simulink model "sm_wing_landing_gear"  (R2021b)
settings: Solver=ode45  StartTime=0  StopTime=10  RelTol=1e-4  AbsTol=1e-4  EnableMultiTasking=on
model workspace (MAT data in the model file):
  ddgrey = [0.15 0.15 0.15]
  dgrey = [0.3 0.3 0.3]
  grey = [0.5 0.5 0.5]
  lgrey = [0.7 0.7 0.7]
  rho_alum = 2700
undefined symbols (not defined in the file): sigbuilder_block, X, Y, Z
libraries: sm_lib x59, sm_wing_landing_gear_lib x45, nesl_utility x7, simulink x2
(part 1 of 3)
Description:
  | Airplane Wing Landing Gear
  | 
  | This model shows a wing landing gear mechanism that can deploy
  | and retract based on the input deploy signal. The mechanism consists
  | of the main column that houses the wheel assembly and the locking
  | mechanism that is used to lock the landing gear in the deployed
  | position.
  | 
  | The mechanism is controlled by two low level controllers (one for
  | deploying and retracting the main column and the other  to lock and
  | unlock the main column into position) and a master controller that
  | coordinates them. The low level controllers are both simple PID
  | controllers. The master controller turns on the deploy/retract
  | controller to deploy the landing gear and when the main column is
  | close enough to the deployed position, it disables the deploy/retract
  |  controller and uses the locking controller to lock the mechanism
  | into position. The reverse happens during retraction.
settings Model: Creator=The MathWorks, Inc.  LastModifiedBy=The MathWorks, Inc.
settings SolverCC: AutoScaleAbsTol=off  AlgebraicLoopSolver=TrustRegion
settings DataIOCC: LimitDataPoints=on  SaveFormat=Array  ReturnWorkspaceOutputs=off
settings OptimizationCC: OptimizeBlockIOStorage=off  BufferReuse=off  GlobalBufferReuse=off  ExpressionFolding=off  ExpressionDepthLimit=2147483647  LocalBlockOutputs=off  LifeSpan=inf  OptimizeDataStoreBuffers=off  BusAssignmentInplaceUpdate=off
settings DebuggingCC: UnderspecifiedInitializationDetection=Classic  MergeDetectMultiDrivingBlocksExec=none  ParameterPrecisionLossMsg=none  FcnCallInpInsideContextMsg=warning  AllowSymbolicDim=off  StateNameClashWarn=warning  SFUnexpectedBacktrackingDiag=warning  SFNoUnconditionalDefaultTransitionDiag=warning  SFExecutionAtInitializationDiag=none  SFMachineParentedDataDiag=warning  ArithmeticOperatorsInVariantConditions=warning
settings HardwareCC: ProdBitPerPointer=32  ProdBitPerSizeT=32  ProdBitPerPtrDiffT=32  ProdLargestAtomicFloat=None  ProdIntDivRoundTo=Undefined  ProdEndianess=Unspecified  ProdWordSize=32  ProdHWDeviceType=32-bit Generic
settings ModelReferenceCC: PropagateSignalLabelsOutOfModel=off
settings SFSimCC: SimUseLocalCustomCode=off  CustomCodeUndefinedFunction=UseInterfaceOnly
settings RTWCC: RTWUseLocalCustomCode=off
settings CodeAppCC: StateflowObjectComments=on
settings GRTTargetCC: TargetLangStandard=C89/C90 (ANSI)  CombineOutputUpdateFcns=off  GRTInterface=on
settings ConfigComp: CovMetricSettings=dw  CovSaveCumulativeToWorkspaceVar=on  CovSaveSingleToWorkspaceVar=on  CovExternalEMLEnable=off  CovSFcnEnable=off
settings SimscapeCC: SimscapeNormalizeSystem=off
settings ConfigurationSet: Description=SimMechanics 2G
settings ExplorerConfigSet: InternalSimMechanicsExplorerSettings="<ExplorerConfiguration><canonicalview>default</canonicalview><AnimationSetting><BasePlaybackSpeed>1.0</BasePlaybackSpeed><PlaybackSpeedFactor>1.0</PlaybackSpeedFactor></AnimationSetting><TilePanel><TileInfo><Tiles Columns=\"1\" Count=\"1\" Rows=\"1\"><Column Left=\"2\" Weight=\"1\"/><Column Left=\"642\"/><Row Top=\"2\" Weight=\"1\"/><Row Top=\"563\"/><Tile Height=\"1\" Width=\"1\" X=\"0\" Y=\"0\"/></Tiles></TileInfo><SceneInfo><SceneViewer><BGColor><R>0.60000002384185791</R><G>0.60000002384185791</G><B>0.60000002384185791</B></BGColor><Camera><Position><X>5.05242413843680716</X><Y>-3.63242412174750484</Y><Z>3.34347951973487101</Z></Position><Center><X>1.82500004768371582</X><Y>-0.405000030994415283</Y><Z>0.116055428981781006</Z></Center><Up><X>-0.408248290463863073</X><Y>0.408248290463863073</Y><Z>0.816496580927726145</Z></Up><Left>-2.13829092979431179</Left><Right>2.13829092979431179</Right><Bottom>-1.76270043253898634</Bottom><Top>1.76270043253898634</Top></Camera></SceneViewer></SceneInfo></TilePanel></ExplorerConfiguration>"

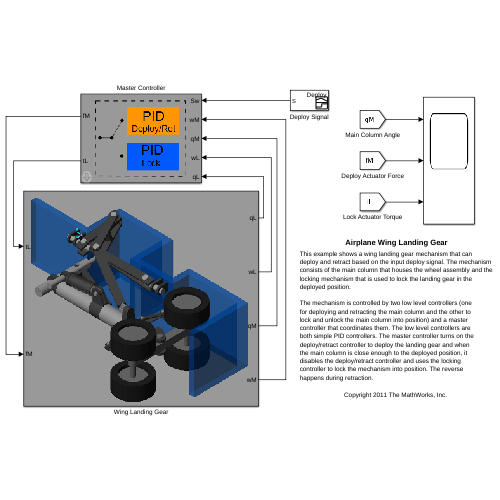
[thumbnail: Simulink's stored preview of the top-level diagram]
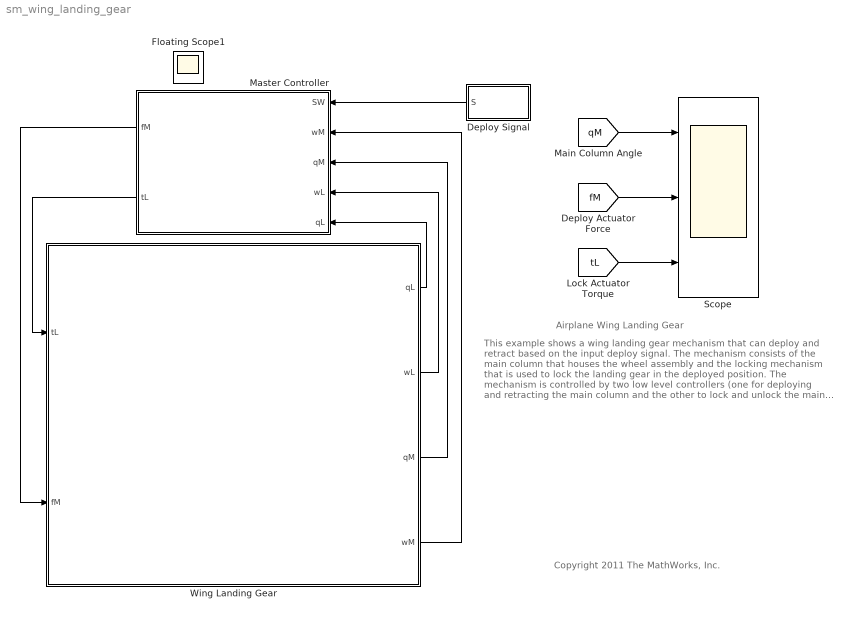
== system sm_wing_landing_gear ==
  note: Airplane Wing Landing Gear
  note: Copyright 2011 The MathWorks, Inc.
  note: This example shows a wing landing gear mechanism that can
      | deploy and retract based on the input deploy signal. The mechanism
      | consists of the main column that houses the wheel assembly and the
      | locking mechanism that is used to lock the landing gear in the
      | deployed position.
      |
      | The mechanism is controlled by two low level controllers (one
      | for deploying and retracting the main column and the other to
      | lock and unlock the main column into position) and a master
      | controller that coordinates them. The low level controllers are
      | both simple PID controllers. The master controller turns on the
      | deploy/retract controller to deploy the landing gear and when
      | the main column is close enough to the deployed position, it
      | disables the deploy/retract controller and uses the locking
      | controller to lock the mechanism into position. The reverse
      | happens during retraction.
  Deploy Signal : Subsystem  Tag=STV Subsys  LoadFcn=sigbuilder_block('load');  StartFcn=sigbuilder_block('start');  StopFcn=sigbuilder_block('stop');  ClipboardFcn=sigbuilder_block('clipboard');  mask(Sigbuilder block){tuvar=[0:10]}
      mask help: Simulink:masks:SigbuilderBlock_MD
      mask init:
      | if ~strcmp(get_param(bdroot(gcbh),'SimulationStatus'),'stopped') tuvar = sigbuilder_block('maskInit'); end
      settings: CopyFcn=sigbuilder_block('copy');  DeleteFcn=sigbuilder_block('delete');  ModelCloseFcn=sigbuilder_block('modelClose');  PreSaveFcn=sigbuilder_block('preSave');  PauseFcn=sigbuilder_block('pause');  ContinueFcn=sigbuilder_block('continue');  NameChangeFcn=sigbuilder_block('namechange');  OpenFcn=sigbuilder_block('open',[387.2 208 550.4 400 ]);  CloseFcn=sigbuilder_block('close');
      mask Display: plot(0, 0, 100, 100,[2, 2, 32, 32, 2], [68, 8, 8, 68, 68],[32, 2], [38, 38], [32, 19, 2],[53, 60, 44], [32, 17, 17, 2],[16, 16, 31, 31]);txt = getActiveGroup(gcbh);text(2, 100, txt,'verticalAlignment', 'top');
  Master Controller : Subsystem  mask(Controller){Kpd=2e5, Kdd=5e4, Kid=10, Kpl=4, Kdl=1, Kil=0.5, qL=5, qUL=1}
      mask prompts: Kpd "Proportional Gain"; Kdd "Derivative Gain"; Kid "Integral Gain"; Kpl "Proportional Gain"; Kdl "Derivative Gain"; Kil "Integral Gain"; qL "Locking Start Angle (deg)"; qUL "Unlocking End Angle (deg)"
      mask help: The mechanism is controlled by two low level controllers (one for deploying and retracting the main column and the other to lock and unlock the main column into position) and a master controller that coordinates them. The low level controllers are both simple PID controllers. The master controller turns on the Deploy/Retract controller which moves the main column into the vertical position. When the angle of the main column is within a certain value of the vertical position (Locking Start Angle specified below), the Locking controller is enabled and the Deploy/Retract Controller is disabled. The Locking controller makes the locking links fully stretched leaving the mechanism in a locked position. During retraction the Locking controller makes the locking links to be bent and starts to lift the main column. Once the main column angle is more than a certain value from the vertical position (Unlocking End Angle specified below), the Locking controller is disabled and the Deploy/Retract controller is enabled, which moves the main column to the horizontal position.
      mask DialogControl ParameterTabVar0 Prompt: Deploy Ctrl
      mask DialogControl ParameterTabVar01 Prompt: Lock Ctrl
      mask DialogControl ParameterTabVar012 Prompt: Master Ctrl
      mask Display:
      | image('sm_wlandgear_controller.png');
      | port_label('input',1,'Sw');
      | port_label('input',2,'wM');
      | port_label('input',3,'qM');
      | port_label('input',4,'wL');
      | port_label('input',5,'qL');
      | port_label('output',2,'tL');
      | port_label('output',1,'fM');
  Scope : Scope  NumInputPorts=3
  Wing Landing Gear : Subsystem
      mask Display:
      | image('sm_wlandgear_plant.png');
      | port_label('output',1,'qL');
      | port_label('output',2,'wL');
      | port_label('output',3,'qM');
      | port_label('output',4,'wM');
      | port_label('input',2,'fM');
      | port_label('input',1,'tL');
  Floating Scope1 : Scope
  wires:
  Deploy Signal/1(S) -> Master Controller/1(SW)
  [tL] -> Scope/3
  [fM] -> Scope/2
  [qM] -> Scope/1
  Wing Landing Gear/1(qL) -> Master Controller/5(qL)
  Wing Landing Gear/2(wL) -> Master Controller/4(wL)
  Wing Landing Gear/3(qM) -> Master Controller/3(qM)
  Wing Landing Gear/4(wM) -> Master Controller/2(wM)
  Master Controller/1(fM) -> Wing Landing Gear/2(fM)
  Master Controller/2(tL) -> Wing Landing Gear/1(tL)

== system sm_wing_landing_gear/Deploy Signal ==
  Demux : Demux  Tag=STV Demux  Outputs=1
      settings: DisplayOption=none
  FromWs : FromWorkspace  Tag=STV FromWs  VariableName=tuvar
      SigBuilderData=|
      | common.afterFinalStr = 'Extrapolate'
      | common.sampleTime = '0'
      | dataSet.timeRange = [0 15]
      | dataSet.name = 'Deploy'
      | sbobj.Groups.Name = 'Deploy'
      | sbobj.Groups.Signals.Name = 'S'
      | sbobj.Groups.Signals.XData = [0 1 1 6 6 15]
      | sbobj.Groups.Signals.YData = [0 0 1 1 0 0]
      | sbobj.Groups.TimeRange = [0 15]
  S : Outport  Tag=STV Outport  VectorParamsAs1DForOutWhenUnconnected=off
  wires:
  Demux/1 -> S/1
  FromWs/1 -> Demux/1

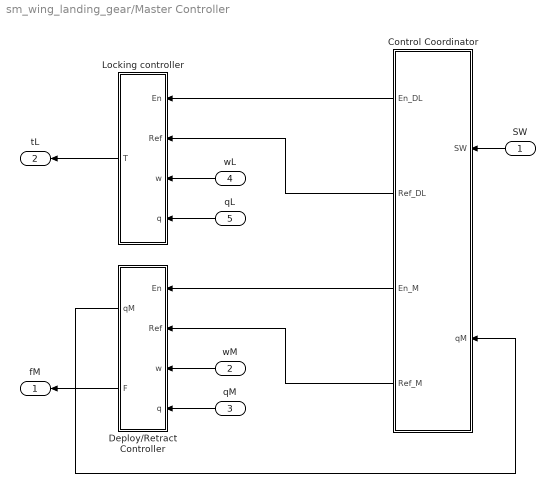
== system sm_wing_landing_gear/Master Controller ==
  SW : Inport
  wM : Inport  Port=2
  qM : Inport  Port=3
  wL : Inport  Port=4
  qL : Inport  Port=5
  Control Coordinator : Subsystem  mask{On_act_ang=qL, lock_tgt=180, Off_act_ang=qUL, unlock_tgt=100}
      mask prompts: On_act_ang "Locking begins when main angle is within (deg)"; lock_tgt "Locking target angle (deg)"; Off_act_ang "Unlocking ends when main is more than angle (deg)"; unlock_tgt "Unlocking target angle (deg)"
  Deploy/Retract Controller : Subsystem  mask{Kp=Kpd, Kd=Kdd, Ki=Kid}
      mask prompts: Kp "Proportional Gain"; Kd "Derivative Gain"; Ki "Integral Gain"
  Locking controller : Subsystem  mask{Kp=Kpl, Kd=Kdl, Ki=Kil}
      mask prompts: Kp "Proportional Gain"; Kd "Derivative Gain"; Ki "Integral Gain"
  fM : Outport  VectorParamsAs1DForOutWhenUnconnected=off
  tL : Outport  Port=2  VectorParamsAs1DForOutWhenUnconnected=off
  wires:
  Control Coordinator/3(En_M) -> Deploy/Retract Controller/1(En)
  Control Coordinator/1(En_DL) -> Locking controller/1(En)
  Control Coordinator/2(Ref_DL) -> Locking controller/2(Ref)
  Control Coordinator/4(Ref_M) -> Deploy/Retract Controller/2(Ref)
  Deploy/Retract Controller/1(qM) -> Control Coordinator/2(qM)
  SW/1 -> Control Coordinator/1(SW)
  Locking controller/1(T) -> tL/1
  wL/1 -> Locking controller/3(w)
  qL/1 -> Locking controller/4(q)
  wM/1 -> Deploy/Retract Controller/3(w)
  qM/1 -> Deploy/Retract Controller/4(q)
  Deploy/Retract Controller/2(F) -> fM/1

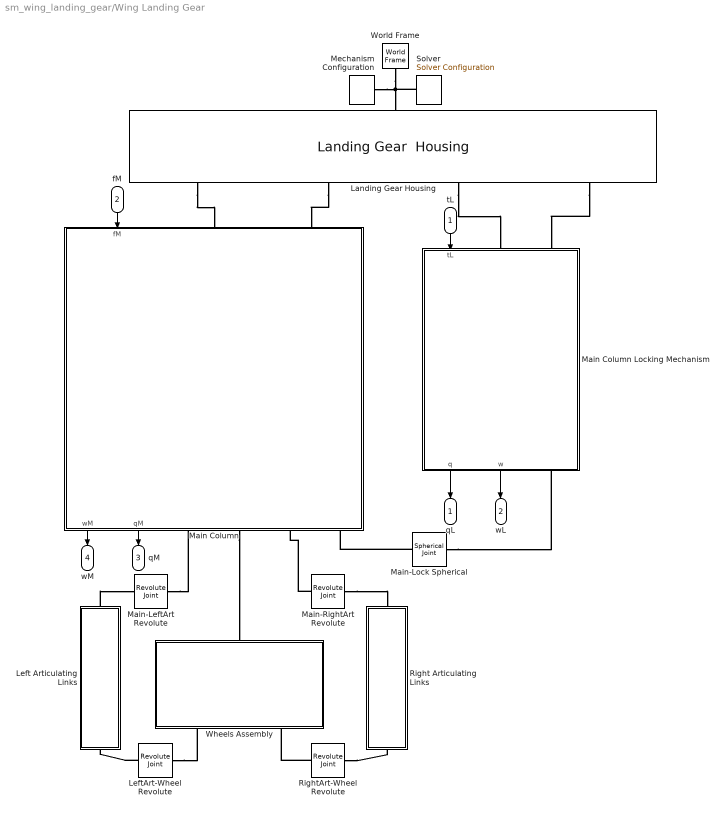
== system sm_wing_landing_gear/Wing Landing Gear ==
  tL : Inport
  fM : Inport  Port=2
  Landing Gear Housing : sm_wing_landing_gear_lib/Landing Gear  Housing  L1=100  L2=60  L3=90  L4=60  L5=70  L6=30  L7=100  L8=100  T=10  H=100  Hb=75  H1=[105 -5 3*60/8-20]  H2=[20 20 0]  H3=[145 40 0]  H4=[-7 40 0]  clr=[0 0.4 0.9]  Op=0.5
      settings: SourceProductBaseCode=MS
  Left Articulating Links : Subsystem
      mask Display:
      | image('sm_wlandgear_artlinks.png');
      | port_label('LConn',1,'B');
      | port_label('RConn',1,'F');
  LeftArt-Wheel Revolute : sm_lib/Joints/Revolute Joint  JointMode=Normal  SenseConstraintForce=off  SenseConstraintForceX=off  SenseConstraintForceY=off  SenseConstraintForceZ=off  SenseConstraintTorque=off  SenseConstraintTorqueX=off  SenseConstraintTorqueY=off  SenseConstraintTorqueZ=off  SenseTotalForce=off  SenseTotalForceX=off  SenseTotalForceY=off  SenseTotalForceZ=off  SenseTotalTorque=off  SenseTotalTorqueX=off  SenseTotalTorqueY=off  SenseTotalTorqueZ=off  CompositeWrenchDir=FollowerOnBase  CompositeWrenchFrame=BaseFrame  EquilibriumPosition=0  EquilibriumPositionUnits=rad  SpringStiffness=0  SpringStiffnessUnits=N*m/rad  DampingCoefficient=0  DampingCoefficientUnits=N*m/(rad/s)  TorqueActuationMode=NoTorque  MotionActuationMode=ComputedMotion  SensePosition=off  SenseVelocity=off  SenseAcceleration=off  SenseTorqueForce=off  SenseLowerLimitTorqueForce=off  SenseUpperLimitTorqueForce=off  LowerLimitSpecify=off  LowerLimitBound=-90  LowerLimitBoundUnits=deg  LowerLimitStiffness=1e4  LowerLimitStiffnessUnits=N*m/deg  LowerLimitDamping=10  LowerLimitDampingUnits=N*m/(deg/s)  LowerLimitTransitionRegionWidth=0.1  LowerLimitTransitionRegionWidthUnits=deg  UpperLimitSpecify=off  UpperLimitBound=90  UpperLimitBoundUnits=deg  UpperLimitStiffness=1e4  UpperLimitStiffnessUnits=N*m/deg  UpperLimitDamping=10  UpperLimitDampingUnits=N*m/(deg/s)  UpperLimitTransitionRegionWidth=0.1  UpperLimitTransitionRegionWidthUnits=deg  PositionTargetSpecify=off  PositionTargetPriority=Low  PositionTargetValue=180  PositionTargetValueUnits=deg  VelocityTargetSpecify=off  VelocityTargetPriority=Low  VelocityTargetValue=0  VelocityTargetValueUnits=rad/s
  Main Column : Subsystem
      mask Display:
      | image('sm_wlandgear_maincolumn.png');
      | port_label('input',1,'fM');
      | port_label('LConn',1,'H1');
      | port_label('LConn',2,'H2');
      | port_label('output',1,'wM');
      | port_label('output',2,'qM');
      | port_label('RConn',1,'AL');
      | port_label('RConn',2,'W');
      | port_label('RConn',3,'AR');
      | port_label('RConn',4,'S');
  Main Column Locking Mechanism : Subsystem
      mask Display:
      | image('sm_wlandgear_lockmechanism.png');
      | port_label('RConn',1,'S');
      | port_label('output',1,'qL');
      | port_label('output',2,'wL');
      | port_label('LConn',1,'H3');
      | port_label('LConn',2,'H4');
      | port_label('input',1,'tL');
  Main-LeftArt Revolute : sm_lib/Joints/Revolute Joint  JointMode=Normal  SenseConstraintForce=off  SenseConstraintForceX=off  SenseConstraintForceY=off  SenseConstraintForceZ=off  SenseConstraintTorque=off  SenseConstraintTorqueX=off  SenseConstraintTorqueY=off  SenseConstraintTorqueZ=off  SenseTotalForce=off  SenseTotalForceX=off  SenseTotalForceY=off  SenseTotalForceZ=off  SenseTotalTorque=off  SenseTotalTorqueX=off  SenseTotalTorqueY=off  SenseTotalTorqueZ=off  CompositeWrenchDir=FollowerOnBase  CompositeWrenchFrame=BaseFrame  EquilibriumPosition=0  EquilibriumPositionUnits=rad  SpringStiffness=0  SpringStiffnessUnits=N*m/rad  DampingCoefficient=0  DampingCoefficientUnits=N*m/(rad/s)  TorqueActuationMode=NoTorque  MotionActuationMode=ComputedMotion  SensePosition=off  SenseVelocity=off  SenseAcceleration=off  SenseTorqueForce=off  SenseLowerLimitTorqueForce=off  SenseUpperLimitTorqueForce=off  LowerLimitSpecify=off  LowerLimitBound=-90  LowerLimitBoundUnits=deg  LowerLimitStiffness=1e4  LowerLimitStiffnessUnits=N*m/deg  LowerLimitDamping=10  LowerLimitDampingUnits=N*m/(deg/s)  LowerLimitTransitionRegionWidth=0.1  LowerLimitTransitionRegionWidthUnits=deg  UpperLimitSpecify=off  UpperLimitBound=90  UpperLimitBoundUnits=deg  UpperLimitStiffness=1e4  UpperLimitStiffnessUnits=N*m/deg  UpperLimitDamping=10  UpperLimitDampingUnits=N*m/(deg/s)  UpperLimitTransitionRegionWidth=0.1  UpperLimitTransitionRegionWidthUnits=deg  PositionTargetSpecify=off  PositionTargetPriority=Low  PositionTargetValue=180  PositionTargetValueUnits=deg  VelocityTargetSpecify=off  VelocityTargetPriority=Low  VelocityTargetValue=0  VelocityTargetValueUnits=rad/s
  Main-Lock Spherical : sm_lib/Joints/Spherical Joint  JointMode=Normal  SenseConstraintForce=off  SenseConstraintForceX=off  SenseConstraintForceY=off  SenseConstraintForceZ=off  SenseConstraintTorque=off  SenseConstraintTorqueX=off  SenseConstraintTorqueY=off  SenseConstraintTorqueZ=off  SenseTotalForce=off  SenseTotalForceX=off  SenseTotalForceY=off  SenseTotalForceZ=off  SenseTotalTorque=off  SenseTotalTorqueX=off  SenseTotalTorqueY=off  SenseTotalTorqueZ=off  CompositeWrenchDir=FollowerOnBase  CompositeWrenchFrame=BaseFrame  DefPosRotationMethod=None  DefPosRotationAngleUnits=deg  DefPosRotationStandardAxis=+Z  DefPosRotationAngle=0  DefPosRotationArbitraryAxis=[0 0 1]  DefPosFollAlignAxisA=+X  DefPosBaseAlignAxisA=+Y  DefPosFollAlignAxisB=+Y  DefPosBaseAlignAxisB=+Z  DefPosRotationSequenceAxes=FollowerAxes  DefPosRotationSequence=XYX  DefPosRotationSequenceAngles=[0 0 0]  DefPosRotationSequenceAnglesUnits=deg  DefPosRotationMatrix=[1 0 0; 0 1 0; 0 0 1]  EqPosRotationMethod=None  EqPosRotationAngleUnits=deg  EqPosRotationStandardAxis=+Z  EqPosRotationAngle=0  EqPosRotationArbitraryAxis=[0 0 1]  EqPosFollAlignAxisA=+X  EqPosBaseAlignAxisA=+Y  EqPosFollAlignAxisB=+Y  EqPosBaseAlignAxisB=+Z  EqPosRotationSequenceAxes=FollowerAxes  EqPosRotationSequence=XYX  EqPosRotationSequenceAngles=[0 0 0]  EqPosRotationSequenceAnglesUnits=deg  EqPosRotationMatrix=[1 0 0; 0 1 0; 0 0 1]  SpringStiffness=0  SpringStiffnessUnits=N*m/rad  DampingCoefficient=0  DampingCoefficientUnits=N*m/(rad/s)  ActuateTorqueX=off  ActuateTorqueY=off  ActuateTorqueZ=off  ActuateTorque=off  TorqueActuationMode=NoTorque  MotionActuationMode=ComputedMotion  ActuationFrame=BaseFrame  SensePosition=off  SenseVelocityX=off  SenseVelocityY=off  SenseVelocityZ=off  SenseVelocity=off  SenseAccelerationX=off  SenseAccelerationY=off  SenseAccelerationZ=off  SenseAcceleration=off  SenseTorqueX=off  SenseTorqueY=off  SenseTorqueZ=off  SenseTorqueForce=off  SenseLowerLimitTorqueMag=off  SenseUpperLimitTorqueMag=off  SensingFrame=BaseFrame  LowerLimitSpecify=off  LowerLimitBound=15  LowerLimitBoundUnits=deg  LowerLimitStiffness=1e4  LowerLimitStiffnessUnits=N*m/deg  LowerLimitDamping=10  LowerLimitDampingUnits=N*m/(deg/s)  LowerLimitTransitionRegionWidth=0.1  LowerLimitTransitionRegionWidthUnits=deg  UpperLimitSpecify=off  UpperLimitBound=45  UpperLimitBoundUnits=deg  UpperLimitStiffness=1e4  UpperLimitStiffnessUnits=N*m/deg  UpperLimitDamping=10  UpperLimitDampingUnits=N*m/(deg/s)  UpperLimitTransitionRegionWidth=0.1  UpperLimitTransitionRegionWidthUnits=deg  PositionTargetRotationMethod=AlignedAxes  PositionTargetRotationAngleUnits=deg  PositionTargetRotationStandardAxis=+Z  PositionTargetRotationAngle=0  PositionTargetRotationArbitraryAxis=[0 0 1]  PositionTargetFollAlignAxisA=+Z  PositionTargetBaseAlignAxisA=-Z  PositionTargetFollAlignAxisB=+Y  PositionTargetBaseAlignAxisB=-Y  PositionTargetRotationSequenceAxes=FollowerAxes  PositionTargetRotationSequence=XYX  PositionTargetRotationSequenceAngles=[0 0 0]  PositionTargetRotationSequenceAnglesUnits=deg  PositionTargetRotationMatrix=[1 0 0; 0 1 0; 0 0 1]  PositionTargetSpecify=off  PositionTargetPriority=Low  VelocityTargetValue=[0 0 0]  VelocityTargetValueUnits=rad/s  VelocityTargetSpecify=off  VelocityTargetPriority=Low  VelocityTargetInFollowerFrame=on
  Main-RightArt Revolute : sm_lib/Joints/Revolute Joint  JointMode=Normal  SenseConstraintForce=off  SenseConstraintForceX=off  SenseConstraintForceY=off  SenseConstraintForceZ=off  SenseConstraintTorque=off  SenseConstraintTorqueX=off  SenseConstraintTorqueY=off  SenseConstraintTorqueZ=off  SenseTotalForce=off  SenseTotalForceX=off  SenseTotalForceY=off  SenseTotalForceZ=off  SenseTotalTorque=off  SenseTotalTorqueX=off  SenseTotalTorqueY=off  SenseTotalTorqueZ=off  CompositeWrenchDir=FollowerOnBase  CompositeWrenchFrame=BaseFrame  EquilibriumPosition=0  EquilibriumPositionUnits=rad  SpringStiffness=0  SpringStiffnessUnits=N*m/rad  DampingCoefficient=0  DampingCoefficientUnits=N*m/(rad/s)  TorqueActuationMode=NoTorque  MotionActuationMode=ComputedMotion  SensePosition=off  SenseVelocity=off  SenseAcceleration=off  SenseTorqueForce=off  SenseLowerLimitTorqueForce=off  SenseUpperLimitTorqueForce=off  LowerLimitSpecify=off  LowerLimitBound=-90  LowerLimitBoundUnits=deg  LowerLimitStiffness=1e4  LowerLimitStiffnessUnits=N*m/deg  LowerLimitDamping=10  LowerLimitDampingUnits=N*m/(deg/s)  LowerLimitTransitionRegionWidth=0.1  LowerLimitTransitionRegionWidthUnits=deg  UpperLimitSpecify=off  UpperLimitBound=90  UpperLimitBoundUnits=deg  UpperLimitStiffness=1e4  UpperLimitStiffnessUnits=N*m/deg  UpperLimitDamping=10  UpperLimitDampingUnits=N*m/(deg/s)  UpperLimitTransitionRegionWidth=0.1  UpperLimitTransitionRegionWidthUnits=deg  PositionTargetSpecify=off  PositionTargetPriority=Low  PositionTargetValue=180  PositionTargetValueUnits=deg  VelocityTargetSpecify=off  VelocityTargetPriority=Low  VelocityTargetValue=0  VelocityTargetValueUnits=rad/s
  Mechanism Configuration : sm_lib/Utilities/Mechanism Configuration  UniformGravity=Constant  GravityVector=[0 0 -9.81]  GravityUnits=m/s^2  LinearizationDelta=0.001  JointModeTransitionNonlinearIterations=2
  Right Articulating Links : Subsystem
      mask Display:
      | image('sm_wlandgear_artlinks.png');
      | port_label('LConn',1,'B');
      | port_label('RConn',1,'F');
  RightArt-Wheel Revolute : sm_lib/Joints/Revolute Joint  JointMode=Normal  SenseConstraintForce=off  SenseConstraintForceX=off  SenseConstraintForceY=off  SenseConstraintForceZ=off  SenseConstraintTorque=off  SenseConstraintTorqueX=off  SenseConstraintTorqueY=off  SenseConstraintTorqueZ=off  SenseTotalForce=off  SenseTotalForceX=off  SenseTotalForceY=off  SenseTotalForceZ=off  SenseTotalTorque=off  SenseTotalTorqueX=off  SenseTotalTorqueY=off  SenseTotalTorqueZ=off  CompositeWrenchDir=FollowerOnBase  CompositeWrenchFrame=BaseFrame  EquilibriumPosition=0  EquilibriumPositionUnits=rad  SpringStiffness=0  SpringStiffnessUnits=N*m/rad  DampingCoefficient=0  DampingCoefficientUnits=N*m/(rad/s)  TorqueActuationMode=NoTorque  MotionActuationMode=ComputedMotion  SensePosition=off  SenseVelocity=off  SenseAcceleration=off  SenseTorqueForce=off  SenseLowerLimitTorqueForce=off  SenseUpperLimitTorqueForce=off  LowerLimitSpecify=off  LowerLimitBound=-90  LowerLimitBoundUnits=deg  LowerLimitStiffness=1e4  LowerLimitStiffnessUnits=N*m/deg  LowerLimitDamping=10  LowerLimitDampingUnits=N*m/(deg/s)  LowerLimitTransitionRegionWidth=0.1  LowerLimitTransitionRegionWidthUnits=deg  UpperLimitSpecify=off  UpperLimitBound=90  UpperLimitBoundUnits=deg  UpperLimitStiffness=1e4  UpperLimitStiffnessUnits=N*m/deg  UpperLimitDamping=10  UpperLimitDampingUnits=N*m/(deg/s)  UpperLimitTransitionRegionWidth=0.1  UpperLimitTransitionRegionWidthUnits=deg  PositionTargetSpecify=off  PositionTargetPriority=Low  PositionTargetValue=180  PositionTargetValueUnits=deg  VelocityTargetSpecify=off  VelocityTargetPriority=Low  VelocityTargetValue=0  VelocityTargetValueUnits=rad/s
  Solver : nesl_utility/Solver Configuration  PhysicalDomain=network_engine_domain  SubClassName=solver  LeftPortType=input  RightPortType=generic  Tones=[]  Harmonics=[]  SimulateNoise=off  Profile=off  UseLocalSampling=off  EnableSwitchedLinearOptims=on  FrequencyDomain=off  UseCCode=off  RelTol=0.001  AbsTol=1e-06  MinStep=1e-09  ToWorkspace=off  RevertToSquareIcSolve=off  NumHomotopyIterations=100  PhasorMode=off  PhasorModeNumHarmonics=1  DoDC=off  ResidualTolerance=1e-9  UseLocalSolver=off  LocalSolverChoice=NE_BACKWARD_EULER_ADVANCER  LocalSolverSampleTime=.001  DoFixedCost=off  MaxNonlinIter=3  MaxModeIter=2  ComputeImpulses=off  ImpulseIterations=2  LinearAlgebra=Sparse  EquationFormulation=NE_TIME_EF  DelaysMemoryBudget=1024  AutomaticFiltering=on  FilteringTimeConstant=0.001  PartitionStorageMethod=AS_NEEDED  PartitionMemoryBudget=1024  PartitionMethod=FAST
      settings: SourceProductBaseCode=PW,SS
  Wheels Assembly : Subsystem
      mask Display:
      | image('sm_wlandgear_wheelassm.png');
      | port_label('LConn',1,'FB');
      | port_label('RConn',1,'T');
      | port_label('LConn',2,'RB');
  World Frame : sm_lib/Frames and Transforms/World Frame
  qL : Outport  VectorParamsAs1DForOutWhenUnconnected=off
  wL : Outport  Port=2  VectorParamsAs1DForOutWhenUnconnected=off
  qM : Outport  Port=3  VectorParamsAs1DForOutWhenUnconnected=off
  wM : Outport  Port=4  VectorParamsAs1DForOutWhenUnconnected=off
  wires:
  tL/1 -> Main Column Locking Mechanism/1(tL)
  fM/1 -> Main Column/1(fM)
  Main Column Locking Mechanism/1(q) -> qL/1
  Main Column Locking Mechanism/2(w) -> wL/1
  Main Column/2(qM) -> qM/1
  Main Column/1(wM) -> wM/1
  connections:
  Landing Gear Housing/RConn1 -- Main Column/LConn1
  Left Articulating Links/LConn1 -- Main-LeftArt Revolute/RConn1
  LeftArt-Wheel Revolute/LConn1 -- Left Articulating Links/RConn1
  Main-RightArt Revolute/RConn1 -- Right Articulating Links/LConn1
  Main-LeftArt Revolute/LConn1 -- Main Column/RConn1
  Main Column/RConn2 -- Wheels Assembly/RConn1
  Main-RightArt Revolute/LConn1 -- Main Column/RConn3
  Main-Lock Spherical/LConn1 -- Main Column/RConn4
  LeftArt-Wheel Revolute/RConn1 -- Wheels Assembly/LConn1
  Landing Gear Housing/RConn2 -- Main Column/LConn2
  Main-Lock Spherical/RConn1 -- Main Column Locking Mechanism/RConn1
  World Frame/RConn1 -- Landing Gear Housing/LConn1 -- Mechanism Configuration/RConn1 -- Solver/RConn1
  RightArt-Wheel Revolute/RConn1 -- Right Articulating Links/RConn1
  RightArt-Wheel Revolute/LConn1 -- Wheels Assembly/LConn2
  Landing Gear Housing/RConn3 -- Main Column Locking Mechanism/LConn1
  Landing Gear Housing/RConn4 -- Main Column Locking Mechanism/LConn2

== system sm_wing_landing_gear/Master Controller/Control Coordinator ==
  SW : Inport
  qM : Inport  Port=2
  Logical Operator2 : Logic  Operator=NOT  AllPortsSameDT=off  OutDataTypeStr=boolean
  Ref Signal : Subsystem
  En_DL : Outport  VectorParamsAs1DForOutWhenUnconnected=off
  Ref_DL : Outport  Port=2  VectorParamsAs1DForOutWhenUnconnected=off
  En_M : Outport  Port=3  VectorParamsAs1DForOutWhenUnconnected=off
  Ref_M : Outport  Port=4  VectorParamsAs1DForOutWhenUnconnected=off
  wires:
  Ref Signal/2(EnDL) -> Logical Operator2/1, En_DL/1
  Ref Signal/1(Ref) -> Ref_DL/1
  Logical Operator2/1 -> En_M/1
  SW/1 -> Ref Signal/1(R), Ref_M/1
  qM/1 -> Ref Signal/2(qM)

== system sm_wing_landing_gear/Master Controller/Deploy//Retract Controller ==
  En : Inport
  Ref : Inport  Port=2
  w : Inport  Port=3
  q : Inport  Port=4
  Controller : Subsystem
  Saturation : Saturate  UpperLimit=1e5  LowerLimit=-1e5
  qM : Outport  VectorParamsAs1DForOutWhenUnconnected=off
  F : Outport  Port=2  VectorParamsAs1DForOutWhenUnconnected=off
  tag scope: fM=global, qM=global
  wires:
  q/1 -> Controller/2(q), qM/1, [qM]
  En/1 -> Controller/Enable
  Ref/1 -> Controller/3(Ref)
  Controller/1(F) -> Saturation/1
  Saturation/1 -> [fM], F/1
  w/1 -> Controller/1(w)

== system sm_wing_landing_gear/Master Controller/Locking controller ==
  En : Inport
  Ref : Inport  Port=2
  w : Inport  Port=3
  q : Inport  Port=4
  Controller : Subsystem
  Saturation : Saturate  UpperLimit=1000  LowerLimit=-1000
  T : Outport  VectorParamsAs1DForOutWhenUnconnected=off
  tag scope: tL=global
  wires:
  Controller/1(T) -> Saturation/1
  En/1 -> Controller/Enable
  Ref/1 -> Controller/3(Ref)
  Saturation/1 -> [tL], T/1
  w/1 -> Controller/1(w)
  q/1 -> Controller/2(q)

== system sm_wing_landing_gear/Wing Landing Gear/Left Articulating Links ==
  Lower Articulating Link : sm_wing_landing_gear_lib/Forked Link  L1=40  L2=5  L3=3  L4=2  L5=6  L6=2  H1=8  H2=4  H3=0.5  H4=2  T=6  rho=rho_alum  clr=dgrey
      settings: SourceProductBaseCode=MS
  Lower Peg : sm_lib/Body Elements/Cylindrical Solid  GraphicAmbientColor=[0.5 0.0 0.0 1.0]  BasedOnType=Density  CenterOfMass=[0 0 0]  CenterOfMassUnits=m  GraphicDiffuseColor=lgrey  CylinderLength=12  CylinderLengthUnits=cm  CylinderRadius=2  CylinderRadiusUnits=cm  Density=rho_alum  DensityUnits=kg/(m^3)  DoExposeReferenceFrame=on  GraphicEmissiveColor=[0.0 0.0 0.0 1.0]  ExportEntireGeometry=off  SerializedFrames=<Frames/>  MarkerShape=Sphere  MarkerSize=10  GraphicType=FromGeometry  InertiaType=CalculateFromGeometry  Mass=1  MassUnits=kg  MomentsOfInertia=[1 1 1]  MomentsOfInertiaUnits=kg*m^2  GraphicOpacity=1.0  ProductsOfInertia=[0 0 0]  ProductsOfInertiaUnits=kg*m^2  GraphicShininess=75  GraphicSpecularColor=[0.5 0.5 0.5 1.0]  GraphicVisPropType=SimpleVisualProperties
  Upper Articulating Link : sm_wing_landing_gear_lib/Forked Link  L1=40  L2=5  L3=3  L4=2  L5=6  L6=2  H1=12  H2=8  H3=0.5  H4=2  T=6  rho=rho_alum  clr=dgrey
      settings: SourceProductBaseCode=MS
  Upper Peg : sm_lib/Body Elements/Cylindrical Solid  GraphicAmbientColor=[0.5 0.0 0.0 1.0]  BasedOnType=Density  CenterOfMass=[0 0 0]  CenterOfMassUnits=m  GraphicDiffuseColor=lgrey  CylinderLength=10  CylinderLengthUnits=cm  CylinderRadius=2  CylinderRadiusUnits=cm  Density=rho_alum  DensityUnits=kg/(m^3)  DoExposeReferenceFrame=on  GraphicEmissiveColor=[0.0 0.0 0.0 1.0]  ExportEntireGeometry=off  SerializedFrames=<Frames/>  MarkerShape=Sphere  MarkerSize=10  GraphicType=FromGeometry  InertiaType=CalculateFromGeometry  Mass=1  MassUnits=kg  MomentsOfInertia=[1 1 1]  MomentsOfInertiaUnits=kg*m^2  GraphicOpacity=1.0  ProductsOfInertia=[0 0 0]  ProductsOfInertiaUnits=kg*m^2  GraphicShininess=75  GraphicSpecularColor=[0.5 0.5 0.5 1.0]  GraphicVisPropType=SimpleVisualProperties
  Upper-Lower Revolute : sm_lib/Joints/Revolute Joint  JointMode=Normal  SenseConstraintForce=off  SenseConstraintForceX=off  SenseConstraintForceY=off  SenseConstraintForceZ=off  SenseConstraintTorque=off  SenseConstraintTorqueX=off  SenseConstraintTorqueY=off  SenseConstraintTorqueZ=off  SenseTotalForce=off  SenseTotalForceX=off  SenseTotalForceY=off  SenseTotalForceZ=off  SenseTotalTorque=off  SenseTotalTorqueX=off  SenseTotalTorqueY=off  SenseTotalTorqueZ=off  CompositeWrenchDir=FollowerOnBase  CompositeWrenchFrame=BaseFrame  EquilibriumPosition=0  EquilibriumPositionUnits=rad  SpringStiffness=0  SpringStiffnessUnits=N*m/rad  DampingCoefficient=0  DampingCoefficientUnits=N*m/(rad/s)  TorqueActuationMode=NoTorque  MotionActuationMode=ComputedMotion  SensePosition=off  SenseVelocity=off  SenseAcceleration=off  SenseTorqueForce=off  SenseLowerLimitTorqueForce=off  SenseUpperLimitTorqueForce=off  LowerLimitSpecify=off  LowerLimitBound=-90  LowerLimitBoundUnits=deg  LowerLimitStiffness=1e4  LowerLimitStiffnessUnits=N*m/deg  LowerLimitDamping=10  LowerLimitDampingUnits=N*m/(deg/s)  LowerLimitTransitionRegionWidth=0.1  LowerLimitTransitionRegionWidthUnits=deg  UpperLimitSpecify=off  UpperLimitBound=90  UpperLimitBoundUnits=deg  UpperLimitStiffness=1e4  UpperLimitStiffnessUnits=N*m/deg  UpperLimitDamping=10  UpperLimitDampingUnits=N*m/(deg/s)  UpperLimitTransitionRegionWidth=0.1  UpperLimitTransitionRegionWidthUnits=deg  PositionTargetSpecify=off  PositionTargetPriority=Low  PositionTargetValue=180  PositionTargetValueUnits=deg  VelocityTargetSpecify=off  VelocityTargetPriority=Low  VelocityTargetValue=0  VelocityTargetValueUnits=rad/s
  U : PMIOPort  Side=Left
  L : PMIOPort  Port=2  Side=Right
  connections:
  L/RConn1 -- Lower Articulating Link/RConn1 -- Lower Peg/RConn1
  Lower Articulating Link/LConn1 -- Upper-Lower Revolute/RConn1
  Upper-Lower Revolute/LConn1 -- Upper Articulating Link/RConn1 -- Upper Peg/RConn1
  Upper Articulating Link/LConn1 -- U/RConn1

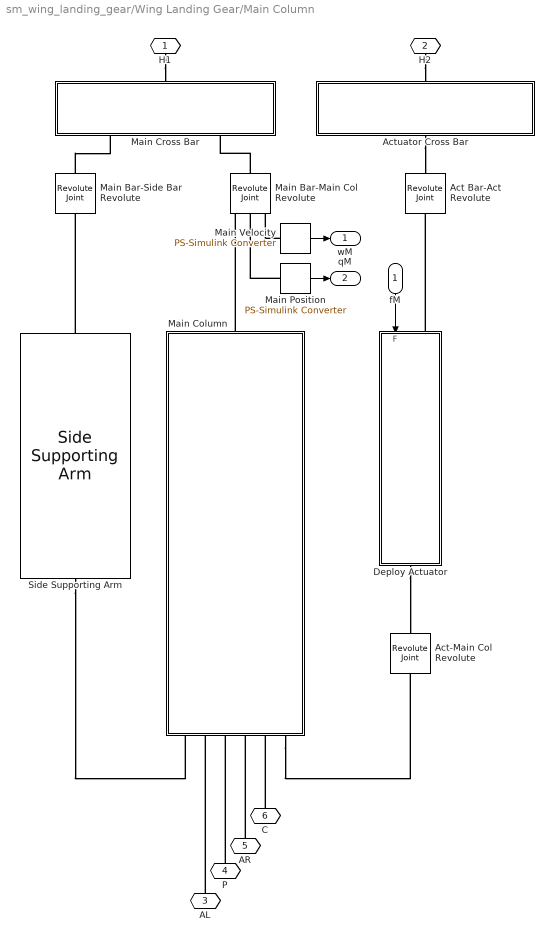
== system sm_wing_landing_gear/Wing Landing Gear/Main Column ==
  fM : Inport
  Act Bar-Act Revolute : sm_lib/Joints/Revolute Joint  JointMode=Normal  SenseConstraintForce=off  SenseConstraintForceX=off  SenseConstraintForceY=off  SenseConstraintForceZ=off  SenseConstraintTorque=off  SenseConstraintTorqueX=off  SenseConstraintTorqueY=off  SenseConstraintTorqueZ=off  SenseTotalForce=off  SenseTotalForceX=off  SenseTotalForceY=off  SenseTotalForceZ=off  SenseTotalTorque=off  SenseTotalTorqueX=off  SenseTotalTorqueY=off  SenseTotalTorqueZ=off  CompositeWrenchDir=FollowerOnBase  CompositeWrenchFrame=BaseFrame  EquilibriumPosition=0  EquilibriumPositionUnits=rad  SpringStiffness=0  SpringStiffnessUnits=N*m/rad  DampingCoefficient=0  DampingCoefficientUnits=N*m/(rad/s)  TorqueActuationMode=NoTorque  MotionActuationMode=ComputedMotion  SensePosition=off  SenseVelocity=off  SenseAcceleration=off  SenseTorqueForce=off  SenseLowerLimitTorqueForce=off  SenseUpperLimitTorqueForce=off  LowerLimitSpecify=off  LowerLimitBound=-90  LowerLimitBoundUnits=deg  LowerLimitStiffness=1e4  LowerLimitStiffnessUnits=N*m/deg  LowerLimitDamping=10  LowerLimitDampingUnits=N*m/(deg/s)  LowerLimitTransitionRegionWidth=0.1  LowerLimitTransitionRegionWidthUnits=deg  UpperLimitSpecify=off  UpperLimitBound=90  UpperLimitBoundUnits=deg  UpperLimitStiffness=1e4  UpperLimitStiffnessUnits=N*m/deg  UpperLimitDamping=10  UpperLimitDampingUnits=N*m/(deg/s)  UpperLimitTransitionRegionWidth=0.1  UpperLimitTransitionRegionWidthUnits=deg  PositionTargetSpecify=off  PositionTargetPriority=Low  PositionTargetValue=0  PositionTargetValueUnits=rad  VelocityTargetSpecify=off  VelocityTargetPriority=Low  VelocityTargetValue=0  VelocityTargetValueUnits=rad/s
  Act-Main Col Revolute : sm_lib/Joints/Revolute Joint  JointMode=Normal  SenseConstraintForce=off  SenseConstraintForceX=off  SenseConstraintForceY=off  SenseConstraintForceZ=off  SenseConstraintTorque=off  SenseConstraintTorqueX=off  SenseConstraintTorqueY=off  SenseConstraintTorqueZ=off  SenseTotalForce=off  SenseTotalForceX=off  SenseTotalForceY=off  SenseTotalForceZ=off  SenseTotalTorque=off  SenseTotalTorqueX=off  SenseTotalTorqueY=off  SenseTotalTorqueZ=off  CompositeWrenchDir=FollowerOnBase  CompositeWrenchFrame=BaseFrame  EquilibriumPosition=0  EquilibriumPositionUnits=rad  SpringStiffness=0  SpringStiffnessUnits=N*m/rad  DampingCoefficient=0  DampingCoefficientUnits=N*m/(rad/s)  TorqueActuationMode=NoTorque  MotionActuationMode=ComputedMotion  SensePosition=off  SenseVelocity=off  SenseAcceleration=off  SenseTorqueForce=off  SenseLowerLimitTorqueForce=off  SenseUpperLimitTorqueForce=off  LowerLimitSpecify=off  LowerLimitBound=-90  LowerLimitBoundUnits=deg  LowerLimitStiffness=1e4  LowerLimitStiffnessUnits=N*m/deg  LowerLimitDamping=10  LowerLimitDampingUnits=N*m/(deg/s)  LowerLimitTransitionRegionWidth=0.1  LowerLimitTransitionRegionWidthUnits=deg  UpperLimitSpecify=off  UpperLimitBound=90  UpperLimitBoundUnits=deg  UpperLimitStiffness=1e4  UpperLimitStiffnessUnits=N*m/deg  UpperLimitDamping=10  UpperLimitDampingUnits=N*m/(deg/s)  UpperLimitTransitionRegionWidth=0.1  UpperLimitTransitionRegionWidthUnits=deg  PositionTargetSpecify=off  PositionTargetPriority=Low  PositionTargetValue=0  PositionTargetValueUnits=rad  VelocityTargetSpecify=off  VelocityTargetPriority=Low  VelocityTargetValue=0  VelocityTargetValueUnits=rad/s
  Actuator Cross Bar : Subsystem
      mask Display:
      | image('sm_wlandgear_actbar.png');
      | port_label('LConn',1,'C');
      | port_label('RConn',1,'H2');
  Deploy Actuator : Subsystem
      mask Display:
      | image('sm_wlandgear_retact.png');
      | port_label('RConn',1,'P');
      | port_label('input',1,'F');
      | port_label('LConn',1,'C');
  Main Cross Bar : Subsystem
      mask Display:
      | image('sm_wlandgear_mainbar.png');
      | port_label('RConn',1,'A');
      | port_label('RConn',2,'B');
      | port_label('LConn',1,'H1');
  Main Bar-Main Col Revolute : sm_lib/Joints/Revolute Joint  JointMode=Normal  SenseConstraintForce=off  SenseConstraintForceX=off  SenseConstraintForceY=off  SenseConstraintForceZ=off  SenseConstraintTorque=off  SenseConstraintTorqueX=off  SenseConstraintTorqueY=off  SenseConstraintTorqueZ=off  SenseTotalForce=off  SenseTotalForceX=off  SenseTotalForceY=off  SenseTotalForceZ=off  SenseTotalTorque=off  SenseTotalTorqueX=off  SenseTotalTorqueY=off  SenseTotalTorqueZ=off  CompositeWrenchDir=FollowerOnBase  CompositeWrenchFrame=BaseFrame  EquilibriumPosition=0  EquilibriumPositionUnits=rad  SpringStiffness=0  SpringStiffnessUnits=N*m/rad  DampingCoefficient=0  DampingCoefficientUnits=N*m/(rad/s)  TorqueActuationMode=NoTorque  MotionActuationMode=ComputedMotion  SensePosition=on  SenseVelocity=on  SenseAcceleration=off  SenseTorqueForce=off  SenseLowerLimitTorqueForce=off  SenseUpperLimitTorqueForce=off  LowerLimitSpecify=off  LowerLimitBound=-90  LowerLimitBoundUnits=deg  LowerLimitStiffness=1e4  LowerLimitStiffnessUnits=N*m/deg  LowerLimitDamping=10  LowerLimitDampingUnits=N*m/(deg/s)  LowerLimitTransitionRegionWidth=0.1  LowerLimitTransitionRegionWidthUnits=deg  UpperLimitSpecify=off  UpperLimitBound=90  UpperLimitBoundUnits=deg  UpperLimitStiffness=1e4  UpperLimitStiffnessUnits=N*m/deg  UpperLimitDamping=10  UpperLimitDampingUnits=N*m/(deg/s)  UpperLimitTransitionRegionWidth=0.1  UpperLimitTransitionRegionWidthUnits=deg  PositionTargetSpecify=off  PositionTargetPriority=Low  PositionTargetValue=90  PositionTargetValueUnits=deg  VelocityTargetSpecify=off  VelocityTargetPriority=Low  VelocityTargetValue=0  VelocityTargetValueUnits=rad/s
  Main Bar-Side Bar Revolute : sm_lib/Joints/Revolute Joint  JointMode=Normal  SenseConstraintForce=off  SenseConstraintForceX=off  SenseConstraintForceY=off  SenseConstraintForceZ=off  SenseConstraintTorque=off  SenseConstraintTorqueX=off  SenseConstraintTorqueY=off  SenseConstraintTorqueZ=off  SenseTotalForce=off  SenseTotalForceX=off  SenseTotalForceY=off  SenseTotalForceZ=off  SenseTotalTorque=off  SenseTotalTorqueX=off  SenseTotalTorqueY=off  SenseTotalTorqueZ=off  CompositeWrenchDir=FollowerOnBase  CompositeWrenchFrame=BaseFrame  EquilibriumPosition=0  EquilibriumPositionUnits=rad  SpringStiffness=0  SpringStiffnessUnits=N*m/rad  DampingCoefficient=0  DampingCoefficientUnits=N*m/(rad/s)  TorqueActuationMode=NoTorque  MotionActuationMode=ComputedMotion  SensePosition=off  SenseVelocity=off  SenseAcceleration=off  SenseTorqueForce=off  SenseLowerLimitTorqueForce=off  SenseUpperLimitTorqueForce=off  LowerLimitSpecify=off  LowerLimitBound=-90  LowerLimitBoundUnits=deg  LowerLimitStiffness=1e4  LowerLimitStiffnessUnits=N*m/deg  LowerLimitDamping=10  LowerLimitDampingUnits=N*m/(deg/s)  LowerLimitTransitionRegionWidth=0.1  LowerLimitTransitionRegionWidthUnits=deg  UpperLimitSpecify=off  UpperLimitBound=90  UpperLimitBoundUnits=deg  UpperLimitStiffness=1e4  UpperLimitStiffnessUnits=N*m/deg  UpperLimitDamping=10  UpperLimitDampingUnits=N*m/(deg/s)  UpperLimitTransitionRegionWidth=0.1  UpperLimitTransitionRegionWidthUnits=deg  PositionTargetSpecify=on  PositionTargetPriority=High  PositionTargetValue=90  PositionTargetValueUnits=deg  VelocityTargetSpecify=off  VelocityTargetPriority=Low  VelocityTargetValue=0  VelocityTargetValueUnits=rad/s
  Main Column : Subsystem
      mask Display:
      | image('sm_wlandgear_maincol.png');
      | port_label('RConn',1,'SB');
      | port_label('RConn',2,'AL');
      | port_label('RConn',3,'P');
      | port_label('RConn',4,'AR');
      | port_label('RConn',5,'C');
      | port_label('RConn',6,'A');
      | port_label('LConn',1,'H');
  Main Position : nesl_utility/PS-Simulink Converter  PhysicalDomain=network_engine_domain  SubClassName=ps_output  LeftPortType=input  RightPortType=output  PseudoPeriodic=off  Frequencies=[]  Unit=deg  AffineConversion=off
      settings: SourceProductBaseCode=PW,SS
  Main Velocity : nesl_utility/PS-Simulink Converter  PhysicalDomain=network_engine_domain  SubClassName=ps_output  LeftPortType=input  RightPortType=output  PseudoPeriodic=off  Frequencies=[]  Unit=deg/s  AffineConversion=off
      settings: SourceProductBaseCode=PW,SS
  Side Supporting Arm : sm_wing_landing_gear_lib/Side Supporting Arm  L=84  W=30  H=12  T=6  Tt=9  Tb=16  Tf=2  Rf=12  Th=4  Oh=9  Rh=3  rho=rho_alum  clr=dgrey
      settings: SourceProductBaseCode=MS
  H1 : PMIOPort  Side=Left
  H2 : PMIOPort  Port=2  Side=Left
  AL : PMIOPort  Port=3  Side=Right
  P : PMIOPort  Port=4  Side=Right
  AR : PMIOPort  Port=5  Side=Right
  C : PMIOPort  Port=6  Side=Right
  wM : Outport  VectorParamsAs1DForOutWhenUnconnected=off
  qM : Outport  Port=2  VectorParamsAs1DForOutWhenUnconnected=off
  wires:
  fM/1 -> Deploy Actuator/1(F)
  Main Velocity/1 -> wM/1
  Main Position/1 -> qM/1
  connections:
  Main Bar-Side Bar Revolute/LConn1 -- Main Cross Bar/RConn1
  Main Bar-Main Col Revolute/LConn1 -- Main Cross Bar/RConn2
  Actuator Cross Bar/LConn1 -- Act Bar-Act Revolute/LConn1
  Main Column/LConn1 -- Main Bar-Main Col Revolute/RConn1
  Side Supporting Arm/LConn1 -- Main Column/RConn1
  Main Column/RConn6 -- Act-Main Col Revolute/LConn1
  Deploy Actuator/LConn1 -- Act Bar-Act Revolute/RConn1
  Deploy Actuator/RConn1 -- Act-Main Col Revolute/RConn1
  Side Supporting Arm/RConn1 -- Main Bar-Side Bar Revolute/RConn1
  H2/RConn1 -- Actuator Cross Bar/RConn1
  H1/RConn1 -- Main Cross Bar/LConn1
  P/RConn1 -- Main Column/RConn3
  C/RConn1 -- Main Column/RConn5
  AL/RConn1 -- Main Column/RConn2
  AR/RConn1 -- Main Column/RConn4
  Main Velocity/LConn1 -- Main Bar-Main Col Revolute/RConn3
  Main Position/LConn1 -- Main Bar-Main Col Revolute/RConn2

== system sm_wing_landing_gear/Wing Landing Gear/Main Column Locking Mechanism ==
  tL : Inport
  Lock Linkage Base Transform : sm_lib/Frames and Transforms/Rigid Transform  TranslationMethod=None  TranslationStandardOffset=0  TranslationLengthUnit=m  TranslationStandardAxis=+Z  TranslationCartesianOffset=[0 0 0]  TranslationROffset=0  TranslationROffsetUnits=m  TranslationZOffset=0  TranslationZOffsetUnits=m  TranslationThetaOffset=0  TranslationThetaOffsetUnits=deg  RotationMethod=StandardAxis  RotationAngleUnits=deg  RotationStandardAxis=+X  RotationAngle=180  RotationArbitraryAxis=[0 0 1]  FollAlignAxisA=+X  BaseAlignAxisA=+Y  FollAlignAxisB=+Y  BaseAlignAxisB=+Z  RotationSequenceAxes=FollowerAxes  RotationSequence=XYX  RotationSequenceAngles=[0 0 0]  RotationSequenceAnglesUnits=deg  RotationMatrix=[1 0 0; 0 1 0; 0 0 1]
  Lock-Sidestay Revolute : sm_lib/Joints/Revolute Joint  JointMode=Normal  SenseConstraintForce=off  SenseConstraintForceX=off  SenseConstraintForceY=off  SenseConstraintForceZ=off  SenseConstraintTorque=off  SenseConstraintTorqueX=off  SenseConstraintTorqueY=off  SenseConstraintTorqueZ=off  SenseTotalForce=off  SenseTotalForceX=off  SenseTotalForceY=off  SenseTotalForceZ=off  SenseTotalTorque=off  SenseTotalTorqueX=off  SenseTotalTorqueY=off  SenseTotalTorqueZ=off  CompositeWrenchDir=FollowerOnBase  CompositeWrenchFrame=BaseFrame  EquilibriumPosition=0  EquilibriumPositionUnits=rad  SpringStiffness=0  SpringStiffnessUnits=N*m/rad  DampingCoefficient=0  DampingCoefficientUnits=N*m/(rad/s)  TorqueActuationMode=NoTorque  MotionActuationMode=ComputedMotion  SensePosition=off  SenseVelocity=off  SenseAcceleration=off  SenseTorqueForce=off  SenseLowerLimitTorqueForce=off  SenseUpperLimitTorqueForce=off  LowerLimitSpecify=off  LowerLimitBound=-90  LowerLimitBoundUnits=deg  LowerLimitStiffness=1e4  LowerLimitStiffnessUnits=N*m/deg  LowerLimitDamping=10  LowerLimitDampingUnits=N*m/(deg/s)  LowerLimitTransitionRegionWidth=0.1  LowerLimitTransitionRegionWidthUnits=deg  UpperLimitSpecify=off  UpperLimitBound=90  UpperLimitBoundUnits=deg  UpperLimitStiffness=1e4  UpperLimitStiffnessUnits=N*m/deg  UpperLimitDamping=10  UpperLimitDampingUnits=N*m/(deg/s)  UpperLimitTransitionRegionWidth=0.1  UpperLimitTransitionRegionWidthUnits=deg  PositionTargetSpecify=on  PositionTargetPriority=Low  PositionTargetValue=110  PositionTargetValueUnits=deg  VelocityTargetSpecify=off  VelocityTargetPriority=Low  VelocityTargetValue=0  VelocityTargetValueUnits=rad/s
  Side Stay Linkage : Subsystem
      mask Display: image('sm_wlandgear_sidestay.png')
  Side Stay Lock Linkage : Subsystem
      mask Display:
      | image('sm_wlandgear_sidestaylock.png');
      | port_label('RConn',1,'F');
      | port_label('output',1,'q');
      | port_label('output',2,'w');
      | port_label('LConn',1,'B');
      | port_label('input',1,'t');
  B : PMIOPort  Side=Left
  LB : PMIOPort  Port=2  Side=Left
  S : PMIOPort  Port=3  Side=Right
  q : Outport  VectorParamsAs1DForOutWhenUnconnected=off
  w : Outport  Port=2  VectorParamsAs1DForOutWhenUnconnected=off
  wires:
  tL/1 -> Side Stay Lock Linkage/1(tL)
  Side Stay Lock Linkage/1(qL) -> q/1
  Side Stay Lock Linkage/2(wL) -> w/1
  connections:
  S/RConn1 -- Side Stay Linkage/RConn1
  B/RConn1 -- Side Stay Linkage/LConn1
  Lock Linkage Base Transform/RConn1 -- Side Stay Lock Linkage/LConn1
  Lock Linkage Base Transform/LConn1 -- LB/RConn1
  Lock-Sidestay Revolute/LConn1 -- Side Stay Lock Linkage/RConn1
  Side Stay Linkage/RConn2 -- Lock-Sidestay Revolute/RConn1

== system sm_wing_landing_gear/Wing Landing Gear/Right Articulating Links ==
  Lower Articulating Link : sm_wing_landing_gear_lib/Forked Link  L1=40  L2=5  L3=3  L4=2  L5=6  L6=2  H1=8  H2=4  H3=0.5  H4=2  T=6  rho=rho_alum  clr=dgrey
      settings: SourceProductBaseCode=MS
  Lower Peg : sm_lib/Body Elements/Cylindrical Solid  GraphicAmbientColor=[0.5 0.0 0.0 1.0]  BasedOnType=Density  CenterOfMass=[0 0 0]  CenterOfMassUnits=m  GraphicDiffuseColor=lgrey  CylinderLength=12  CylinderLengthUnits=cm  CylinderRadius=2  CylinderRadiusUnits=cm  Density=rho_alum  DensityUnits=kg/(m^3)  DoExposeReferenceFrame=on  GraphicEmissiveColor=[0.0 0.0 0.0 1.0]  ExportEntireGeometry=off  SerializedFrames=<Frames/>  MarkerShape=Sphere  MarkerSize=10  GraphicType=FromGeometry  InertiaType=CalculateFromGeometry  Mass=1  MassUnits=kg  MomentsOfInertia=[1 1 1]  MomentsOfInertiaUnits=kg*m^2  GraphicOpacity=1.0  ProductsOfInertia=[0 0 0]  ProductsOfInertiaUnits=kg*m^2  GraphicShininess=75  GraphicSpecularColor=[0.5 0.5 0.5 1.0]  GraphicVisPropType=SimpleVisualProperties
  Upper Articulating Link : sm_wing_landing_gear_lib/Forked Link  L1=40  L2=5  L3=3  L4=2  L5=6  L6=2  H1=12  H2=8  H3=0.5  H4=2  T=6  rho=rho_alum  clr=dgrey
      settings: SourceProductBaseCode=MS
  Upper Peg : sm_lib/Body Elements/Cylindrical Solid  GraphicAmbientColor=[0.5 0.0 0.0 1.0]  BasedOnType=Density  CenterOfMass=[0 0 0]  CenterOfMassUnits=m  GraphicDiffuseColor=lgrey  CylinderLength=10  CylinderLengthUnits=cm  CylinderRadius=2  CylinderRadiusUnits=cm  Density=rho_alum  DensityUnits=kg/(m^3)  DoExposeReferenceFrame=on  GraphicEmissiveColor=[0.0 0.0 0.0 1.0]  ExportEntireGeometry=off  SerializedFrames=<Frames/>  MarkerShape=Sphere  MarkerSize=10  GraphicType=FromGeometry  InertiaType=CalculateFromGeometry  Mass=1  MassUnits=kg  MomentsOfInertia=[1 1 1]  MomentsOfInertiaUnits=kg*m^2  GraphicOpacity=1.0  ProductsOfInertia=[0 0 0]  ProductsOfInertiaUnits=kg*m^2  GraphicShininess=75  GraphicSpecularColor=[0.5 0.5 0.5 1.0]  GraphicVisPropType=SimpleVisualProperties
  Upper-Lower Revolute : sm_lib/Joints/Revolute Joint  JointMode=Normal  SenseConstraintForce=off  SenseConstraintForceX=off  SenseConstraintForceY=off  SenseConstraintForceZ=off  SenseConstraintTorque=off  SenseConstraintTorqueX=off  SenseConstraintTorqueY=off  SenseConstraintTorqueZ=off  SenseTotalForce=off  SenseTotalForceX=off  SenseTotalForceY=off  SenseTotalForceZ=off  SenseTotalTorque=off  SenseTotalTorqueX=off  SenseTotalTorqueY=off  SenseTotalTorqueZ=off  CompositeWrenchDir=FollowerOnBase  CompositeWrenchFrame=BaseFrame  EquilibriumPosition=0  EquilibriumPositionUnits=rad  SpringStiffness=0  SpringStiffnessUnits=N*m/rad  DampingCoefficient=0  DampingCoefficientUnits=N*m/(rad/s)  TorqueActuationMode=NoTorque  MotionActuationMode=ComputedMotion  SensePosition=off  SenseVelocity=off  SenseAcceleration=off  SenseTorqueForce=off  SenseLowerLimitTorqueForce=off  SenseUpperLimitTorqueForce=off  LowerLimitSpecify=off  LowerLimitBound=-90  LowerLimitBoundUnits=deg  LowerLimitStiffness=1e4  LowerLimitStiffnessUnits=N*m/deg  LowerLimitDamping=10  LowerLimitDampingUnits=N*m/(deg/s)  LowerLimitTransitionRegionWidth=0.1  LowerLimitTransitionRegionWidthUnits=deg  UpperLimitSpecify=off  UpperLimitBound=90  UpperLimitBoundUnits=deg  UpperLimitStiffness=1e4  UpperLimitStiffnessUnits=N*m/deg  UpperLimitDamping=10  UpperLimitDampingUnits=N*m/(deg/s)  UpperLimitTransitionRegionWidth=0.1  UpperLimitTransitionRegionWidthUnits=deg  PositionTargetSpecify=off  PositionTargetPriority=Low  PositionTargetValue=180  PositionTargetValueUnits=deg  VelocityTargetSpecify=off  VelocityTargetPriority=Low  VelocityTargetValue=0  VelocityTargetValueUnits=rad/s
  U : PMIOPort  Side=Left
  L : PMIOPort  Port=2  Side=Right
  connections:
  Upper Articulating Link/LConn1 -- U/RConn1
  Upper Peg/RConn1 -- Upper Articulating Link/RConn1 -- Upper-Lower Revolute/LConn1
  Lower Articulating Link/LConn1 -- Upper-Lower Revolute/RConn1
  Lower Peg/RConn1 -- Lower Articulating Link/RConn1 -- L/RConn1
